simulink model "Subsitemas_Completos"  (R2023b)
settings: Solver=VariableStepAuto  StartTime=0.0  StopTime=10.0  RelTol=1e-3
libraries: simulink x8
settings Model: Creator=marqu  LastModifiedBy=marqu
settings OptimizationCC: ReuseModelBlockBuffer=off

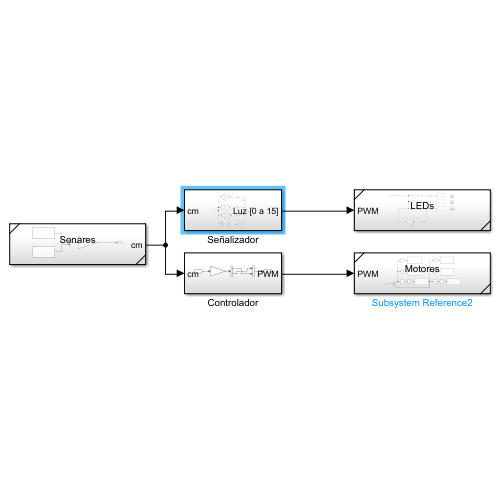
[thumbnail: Simulink's stored preview of the top-level diagram]
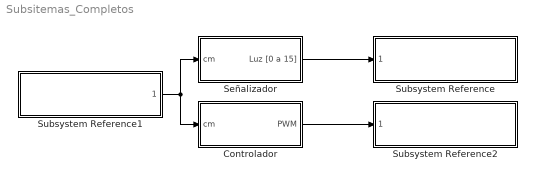
== system Subsitemas_Completos ==
  Controlador : Subsystem
  Señalizador : Subsystem
  Subsystem Reference : Subsystem  ReferencedSubsystem=LEDs
  Subsystem Reference1 : Subsystem  ReferencedSubsystem=Sonares
  Subsystem Reference2 : Subsystem  ReferencedSubsystem=Motores
  wires:
  Controlador/1(PWM) -> Subsystem Reference2/1
  Señalizador/1(Luz [0 a 15]) -> Subsystem Reference/1
  Subsystem Reference1/1 -> Controlador/1(cm), Señalizador/1(cm)

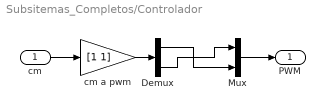
== system Subsitemas_Completos/Controlador ==
  cm : Inport
  Demux : Demux  Outputs=2
  Mux : Mux  Inputs=2
  cm a pwm : Gain  Gain=[1 1]
  PWM : Outport
  wires:
  cm/1 -> cm a pwm/1
  Mux/1 -> PWM/1
  cm a pwm/1 -> Demux/1
  Demux/1 -> Mux/2
  Demux/2 -> Mux/1

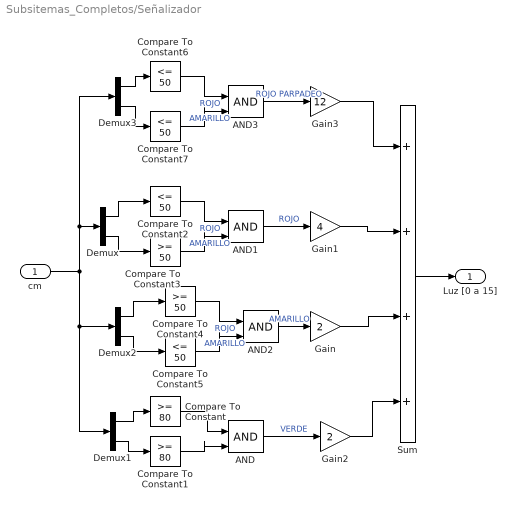
== system Subsitemas_Completos/Señalizador ==
  cm : Inport
  AND{,1..3} (4 alike) : Logic  IconShape=distinctive  AllPortsSameDT=off  OutDataTypeStr=boolean
  Compare To Constant : simulink/Logic and Bit Operations/Compare To Constant  relop=>=  const=80  OutDataTypeStr=boolean
  Compare To Constant1 : simulink/Logic and Bit Operations/Compare To Constant  relop=>=  const=80  OutDataTypeStr=boolean
  Compare To Constant{2,5..7} (4 alike) : simulink/Logic and Bit Operations/Compare To Constant  relop=<=  const=50  OutDataTypeStr=boolean
  Compare To Constant3 : simulink/Logic and Bit Operations/Compare To Constant  relop=>=  const=50  OutDataTypeStr=boolean
  Compare To Constant4 : simulink/Logic and Bit Operations/Compare To Constant  relop=>=  const=50  OutDataTypeStr=boolean
  Demux{,1..3} (4 alike) : Demux  Outputs=2
  Gain : Gain  Gain=2
  Gain1 : Gain  Gain=4
  Gain2 : Gain  Gain=2
  Gain3 : Gain  Gain=12
  Sum : Sum  Inputs=++++
  Luz [0 a 15] : Outport
  wires:
  cm/1 -> Demux1/1, Demux2/1, Demux3/1, Demux/1
  Demux1/2 -> Compare To Constant1/1
  Demux1/1 -> Compare To Constant/1
  Compare To Constant/1 -> AND/1
  Compare To Constant1/1 -> AND/2
  Demux/1 -> Compare To Constant2/1
  Compare To Constant2/1 -> AND1/1  "ROJO"
  AND/1 -> Gain2/1  "VERDE"
  Demux/2 -> Compare To Constant3/1
  Compare To Constant3/1 -> AND1/2  "AMARILLO"
  Compare To Constant5/1 -> AND2/2  "AMARILLO"
  Demux2/1 -> Compare To Constant4/1
  Demux2/2 -> Compare To Constant5/1
  Compare To Constant4/1 -> AND2/1  "ROJO"
  AND2/1 -> Gain/1  "AMARILLO"
  AND1/1 -> Gain1/1  "ROJO"
  Compare To Constant7/1 -> AND3/2  "AMARILLO"
  Demux3/1 -> Compare To Constant6/1
  Demux3/2 -> Compare To Constant7/1
  Compare To Constant6/1 -> AND3/1  "ROJO"
  AND3/1 -> Gain3/1  "ROJO PARPADEO"
  Gain3/1 -> Sum/1
  Gain1/1 -> Sum/2
  Gain/1 -> Sum/3
  Gain2/1 -> Sum/4
  Sum/1 -> Luz [0 a 15]/1
